simulink model "usmernovac"  (Simulink 8.0)
settings: Solver=ode1  StartTime=0.0  StopTime=0.1  FixedStep=1e-6  RelTol=1e-3
undefined symbols (not defined in the file): plecsedit
settings Model: Creator=Kasi  LastModifiedBy=Kasi

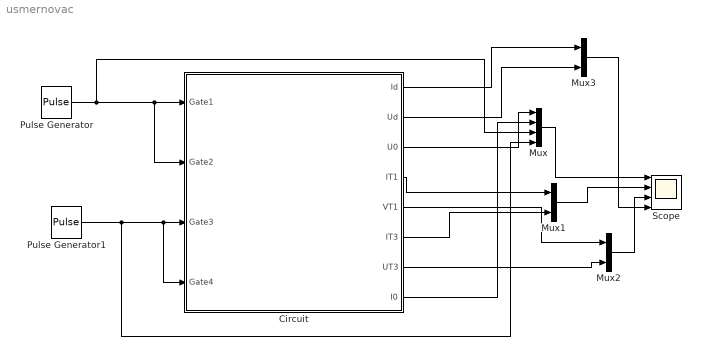
== system usmernovac ==
  Circuit : Subsystem  LoadFcn=plecsedit('sl', 200);  InitFcn=plecsedit('sl', 214);  StartFcn=plecsedit('sl', 208);  StopFcn=plecsedit('sl', 209);  mask(PlecsCircuit){}
      mask init:
      | plecsedit('sl', 200);
      | 
      | % PLACE CUSTOM INITIALIZATIONS ABOVE
      | % DO NOT REMOVE
      | plecsedit('sl', 215);
      | % DO NOT REMOVE
      settings: CopyFcn=plecsedit('sl', 203);  DeleteFcn=plecsedit('sl', 205);  UndoDeleteFcn=plecsedit('sl', 206);  PreSaveFcn=plecsedit('sl', 211);  PostSaveFcn=plecsedit('sl', 201);  NameChangeFcn=plecsedit('sl', 210);  DestroyFcn=plecsedit('sl', 207);  PreCopyFcn=plecsedit('sl', 216);  OpenFcn=plecsedit('sl', 202);  ErrorFcn=plerrorfcn
      mask Display: disp('PLECS\nCircuit')
  Mux : Mux
  Mux1 : Mux  Inputs=2
  Mux2 : Mux  Inputs=2
  Mux3 : Mux  Inputs=2
  Pulse Generator : DiscretePulseGenerator  PulseType=Time based  Amplitude=10  Period=1/50  PulseWidth=5  PhaseDelay=((1/50)/4)/2
  Pulse Generator1 : DiscretePulseGenerator  PulseType=Time based  Amplitude=10  Period=1/50  PulseWidth=5  PhaseDelay=(((1/50)/4)/2)*5
  Scope : Scope  NumInputPorts=4
      settings: YMin=-10~-10~-8~-10  YMax=10~10~8~10
  wires:
  Mux/1 -> Scope/1
  Pulse Generator1/1 -> Mux/4, Circuit/4(Gate4), Circuit/3(Gate3)
  Mux3/1 -> Scope/4
  Pulse Generator/1 -> Mux/3, Circuit/2(Gate2), Circuit/1(Gate1)
  Circuit/4(IT1) -> Mux1/1
  Mux1/1 -> Scope/2
  Circuit/5(VT1) -> Mux2/1
  Mux2/1 -> Scope/3
  Circuit/1(Id) -> Mux3/1
  Circuit/2(Ud) -> Mux3/2
  Circuit/3(U0) -> Mux/1
  Circuit/8(I0) -> Mux/2
  Circuit/6(IT3) -> Mux1/2
  Circuit/7(UT3) -> Mux2/2

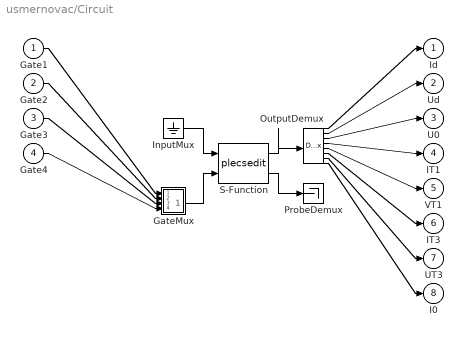
== system usmernovac/Circuit ==
  Gate1 : Inport  PortDimensions=1
  Gate2 : Inport  Port=2  PortDimensions=1
  Gate3 : Inport  Port=3  PortDimensions=1
  Gate4 : Inport  Port=4  PortDimensions=1
  " GateMux " : Subsystem
      mask Display: disp('Mux')
  " InputMux " : Ground
  " OutputDemux " : Demux  Outputs=[ 1 1 1 1 1 1 1 1 ]
  " ProbeDemux " : Terminator
  " S-Function " : S-Function  FunctionName=plecsedit  EnableBusSupport=off
  Id : Outport  PortDimensions=1
  Ud : Outport  Port=2  PortDimensions=1
  U0 : Outport  Port=3  PortDimensions=1
  IT1 : Outport  Port=4  PortDimensions=1
  VT1 : Outport  Port=5  PortDimensions=1
  IT3 : Outport  Port=6  PortDimensions=1
  UT3 : Outport  Port=7  PortDimensions=1
  I0 : Outport  Port=8  PortDimensions=1
  wires:
  " S-Function "/1 -> " OutputDemux "/1
  " InputMux "/1 -> " S-Function "/1
  " GateMux "/1(Out) -> " S-Function "/2
  " S-Function "/2 -> " ProbeDemux "/1
  Gate1/1 -> " GateMux "/1(In1)
  Gate2/1 -> " GateMux "/2(In2)
  Gate3/1 -> " GateMux "/3(In3)
  Gate4/1 -> " GateMux "/4(In4)
  " OutputDemux "/1 -> Id/1
  " OutputDemux "/2 -> Ud/1
  " OutputDemux "/3 -> U0/1
  " OutputDemux "/4 -> IT1/1
  " OutputDemux "/5 -> VT1/1
  " OutputDemux "/6 -> IT3/1
  " OutputDemux "/7 -> UT3/1
  " OutputDemux "/8 -> I0/1

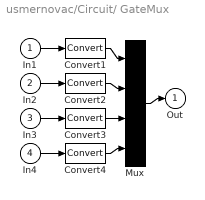
== system usmernovac/Circuit/ GateMux  ==
  In1 : Inport
  In2 : Inport  Port=2
  In3 : Inport  Port=3
  In4 : Inport  Port=4
  Convert{1..4} (4 alike) : DataTypeConversion  SaturateOnIntegerOverflow=on  RndMeth=Zero
  Mux : Mux  Inputs=[ 1 1 1 1 ]
  Out : Outport
  wires:
  Mux/1 -> Out/1
  In1/1 -> Convert1/1
  In2/1 -> Convert2/1
  In3/1 -> Convert3/1
  In4/1 -> Convert4/1
  Convert1/1 -> Mux/1
  Convert2/1 -> Mux/2
  Convert3/1 -> Mux/3
  Convert4/1 -> Mux/4
